simulink model "Simulacion"  (R2025a)
settings: Solver=FixedStepDiscrete  StartTime=0.0  StopTime=1  RelTol=1e-3
libraries: commdigbbndfm2 x2, commchan3 x1, commsink2 x1, commrandsrc3 x1
settings Model: NumberOfSteps=2  Creator=Ruth Juana  LastModifiedBy=Bremdow

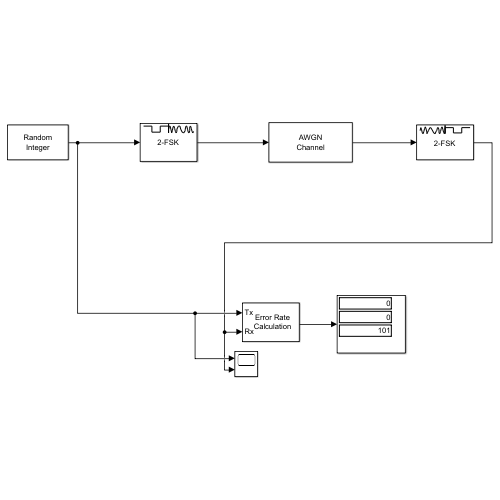
[thumbnail: Simulink's stored preview of the top-level diagram]
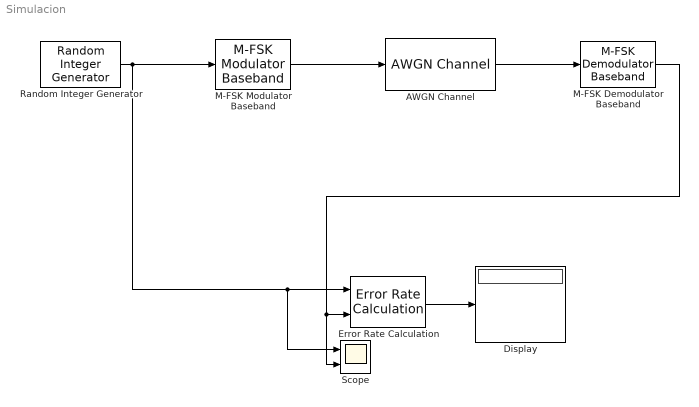
== system Simulacion ==
  AWGN Channel : commchan3/AWGN Channel  LegacyMode=off  NoiseMethod="Signal to noise ratio  (Eb/No)"  noiseMode="Signal to noise ratio  (SNR)"  EbNo=20  EsNo=10  SNR=10  BitsPerSymbol=1  SignalPower=1  SpecifySymbolPeriod=on  SamplesPerSymbol=1  SymbolPeriod=1/1000  VarianceSource=Parameter  Variance=1  RandomStream=Global stream  Seed=67  SimulateUsing=Code generation
  Display : Display
  Error Rate Calculation : commsink2/Error Rate Calculation  N=0  st_delay=0  cp_mode=Entire frame  subframe=[]  PMode=Port  WsName=BeR_Data  RsMode2=off  stop=off  numErr=100  maxBits=1e6
      settings: LibrarySourceBlock=|
      | commhdlsink/Error Rate
      | Calculation
  M-FSK Demodulator Baseband : commdigbbndfm2/M-FSK Demodulator Baseband  M=2  OutType=Integer  Dec=Gray  freqSep=500  numSamp=100  RateOptions=Enforce single-rate processing  outDataType=double
  M-FSK Modulator Baseband : commdigbbndfm2/M-FSK Modulator Baseband  M=2  InType=Integer  Enc=Gray  freqSep=500  phaseType=Continuous  numSamp=100  RateOptions=Enforce single-rate processing  outDataType=double
  Random Integer Generator : commrandsrc3/Random Integer Generator  SetSize=2  SeedSource=Auto  Seed=0  SampleTime=0.01  SamplesPerFrame=1  OutputDataType=double  SimulateUsing=Interpreted execution
  Scope : Scope  NumInputPorts=2
      settings: ActiveDisplayYMinimum=0.33129820051413883  ActiveDisplayYMaximum=0.95629820051413883
  wires:
  Random Integer Generator/1 -> Scope/1, Error Rate Calculation/1, M-FSK Modulator Baseband/1
  M-FSK Modulator Baseband/1 -> AWGN Channel/1
  AWGN Channel/1 -> M-FSK Demodulator Baseband/1
  M-FSK Demodulator Baseband/1 -> Scope/2, Error Rate Calculation/2
  Error Rate Calculation/1 -> Display/1
